simulink model "first_cl_step"  (R2021a)
settings: Solver=VariableStepAuto  StartTime=0.0  StopTime=10  RelTol=1e-3
values from neighbouring files (symbols this model uses):
  K = lqr(sys,Q,R)    [ex2main.m]
  params = get_params()    [ex2main.m]
  sys = get_fullstate_system(params)    [ex2main.m]
settings Model: Creator=martijndebeuf  LastModifiedBy=martijndebeuf
settings SolverCC: AlgebraicLoopSolver=TrustRegion
settings DebuggingCC: SFMachineParentedDataDiag=warning

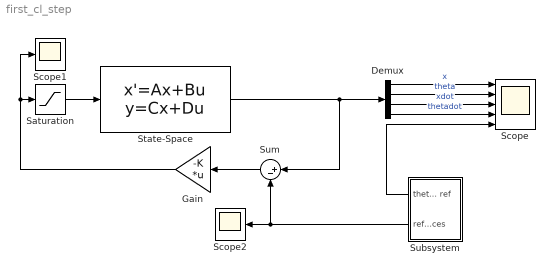
== system first_cl_step ==
  Demux : Demux
  Gain : Gain  Gain=-K  Multiplication=Matrix(K*u) (u vector)
  Saturation : Saturate  UpperLimit=3.5  LowerLimit=-3.5
  Scope : Scope  NumInputPorts=5
  Scope1 : Scope
  Scope2 : Scope
  State-Space : StateSpace  A=sys.A  B=sys.B  C=eye(4)  D=zeros(4,1)  InitialCondition=initial_conditions'
  Subsystem : Subsystem
  Sum : Sum  Inputs=|+-
  wires:
  Sum/1 -> Gain/1
  State-Space/1 -> Demux/1, Sum/1
  Demux/1 -> Scope/1  "x"
  Demux/2 -> Scope/2  "theta"
  Demux/3 -> Scope/3  "xdot"
  Demux/4 -> Scope/4  "thetadot"
  Saturation/1 -> State-Space/1
  Gain/1 -> Scope1/1, Saturation/1
  Subsystem/2(references) -> Sum/2, Scope2/1
  Subsystem/1(theta ref) -> Scope/5

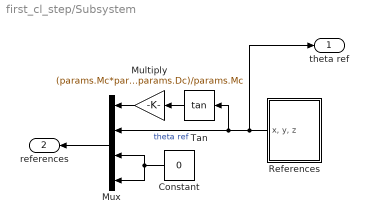
== system first_cl_step/Subsystem ==
  Constant : Constant  Value=0
  Multiply : Gain  Gain=(params.Mc*params.Dt+params.Msw*params.Dc)/params.Mc
  Mux : Mux
  References : Subsystem
  Tan : Trigonometry  Operator=tan
  theta ref : Outport
  references : Outport  Port=2
  wires:
  Mux/1 -> references/1
  Tan/1 -> Multiply/1
  Multiply/1 -> Mux/1
  References/1("x, y, z") -> theta ref/1, Tan/1, Mux/2  "theta ref"
  Constant/1 -> Mux/4, Mux/3

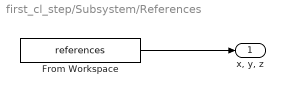
== system first_cl_step/Subsystem/References ==
  From Workspace : FromWorkspace  VariableName=references  SampleTime=0.1  Interpolate=off  OutputAfterFinalValue=Holding final value
  "x, y, z" : Outport
  wires:
  From Workspace/1 -> "x, y, z"/1
